simulink model "Vehicle_Powertrain_Trans_and_Controller_LIB"  (R2014a)
settings: Solver=ode45  StartTime=0.0  StopTime=10.0  RelTol=1e-3
undefined symbols (not defined in the file): clutchRise, p0, pressThresh
libraries: sdl_lib x7, fl_lib x6, nesl_utility x5
Description:
  | Copyright 2014 The MathWorks, Inc.
settings Model: Creator=smiller  LastModifiedBy=smiller
settings DataIOCC: SignalLoggingSaveFormat=ModelDataLogs
settings OptimizationCC: ExpressionDepthLimit=2147483647  InitFltsAndDblsToZero=on
settings DebuggingCC: UnderspecifiedInitializationDetection=Classic  FcnCallInpInsideContextMsg=UseLocalSettings  StateNameClashWarn=warning
settings SFSimCC: SimParseCustomCode=off
settings GRTTargetCC: CombineOutputUpdateFcns=off  GRTInterface=on

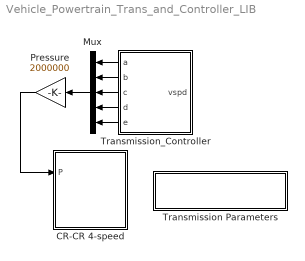
== system Vehicle_Powertrain_Trans_and_Controller_LIB ==
  CR-CR 4-speed : Subsystem  mask(CR-CR 4-Speed){}
      mask help: This is a template for a CR-CR 4-speed transmission. Copy it to your model, open it as a subsystem, and modify it for your use.
      mask init:
      | drive_preinitmask(); Icon = drive_crcrgearblock('Mask');
      settings: OpenFcn=open_system(gcbh,'force');
      mask Help: web(drive_help);
      mask Display:
      | plot(Icon.x1,Icon.y1);
      | plot(Icon.x1_1,Icon.y1_1);
      | plot(Icon.x2,Icon.y2);
      | plot(Icon.x3,Icon.y3);
      | plot(Icon.x3_1,Icon.y3_1);
      | plot(Icon.x4,Icon.y4);
      | plot(Icon.x5,Icon.y5);
      | plot(Icon.x6,Icon.y6);
      | plot(Icon.x7,Icon.y7);
      | plot(Icon.x8,Icon.y8);
      | plot(Icon.x9,Icon.y9);
      | plot(Icon.x10,Icon.y10);
      | plot(Icon.x11,Icon.y11);
      | plot(Icon.x12,Icon.y12);
      | plot(Icon.x13,Icon.y13);
      | plot(Icon.x14,Icon.y14);
      | plot(Icon.x15,Icon.y15);
      | plot(Icon.x16,Icon.y16);
      | plot(Icon.x16_1,Icon.y16_1);
      | plot(Icon.x16_2,Icon.y16_2);
      | plot(Icon.x17,Icon.y17);
      | plot(Icon.x18,Icon.y18);
      | plot(Icon.x18_1,Icon.y18_1);
      | plot(Icon.x18_2,Icon.y18_2);
      | plot(Icon.x19,Icon.y19);
      | plot(Icon.x20,Icon.y20);
      | plot(Icon.x21,Icon.y21);
      | plot(Icon.x22,Icon.y22);
      | plot(Icon.x23,Icon.y23);
      | plot(Icon.x24,Icon.y24);
      | plot(Icon.x25,Icon.y25);
      | plot(Icon.x26,Icon.y26);
      | plot(Icon.x27,Icon.y27);
      | plot(Icon.x28,Icon.y28);
      | plot(Icon.x29,Icon.y29);
      | 
      | plot(Icon.LowerLeftx,Icon.LowerLefty);
      | plot(Icon.UpperRightx,Icon.UpperRighty);
  Mux : Mux  Inputs=5
  Pressure : Gain  Gain=2000000
  Transmission Parameters : Subsystem
      settings: OpenFcn=|
      | num_fric_surf = 6;
      | eff_tor_rad = 0.4;
      | engagement_area = 0.0025;
      | peak_normal = 0.55;
      | fric_coeff = 0.5;
      | clutchRise = 0.1;
      | velTol = 1e-3;
      | pressThresh = 0.05;
      | p0 = 20e5;
      mask Display: fprintf('Double-Click to Define\nTransmission Parameters');
  Transmission_Controller : Stateflow chart  TreatAsAtomicUnit=on
  wires:
  Transmission_Controller/1(a) -> Mux/1
  Transmission_Controller/2(b) -> Mux/2
  Transmission_Controller/3(c) -> Mux/3
  Transmission_Controller/4(d) -> Mux/4
  Transmission_Controller/5(e) -> Mux/5
  Mux/1 -> Pressure/1
  Pressure/1 -> CR-CR 4-speed/1(P)

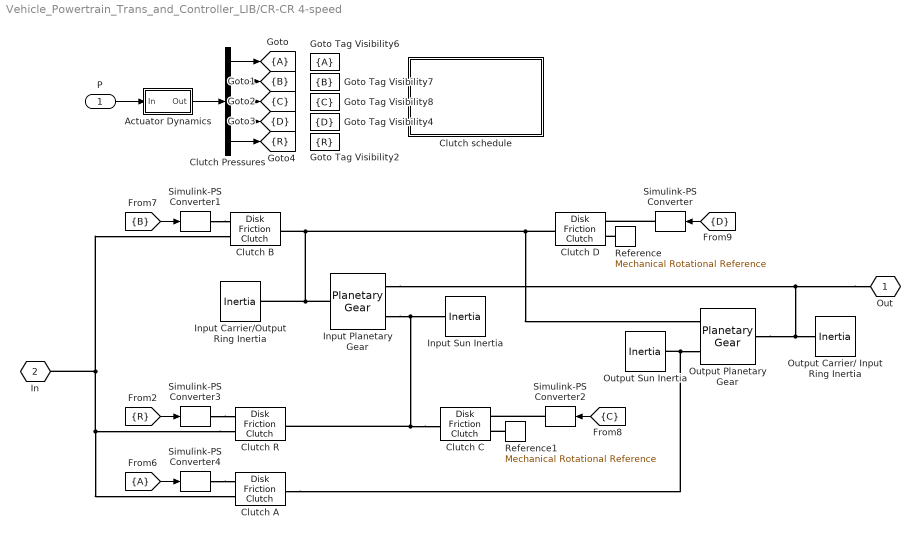
== system Vehicle_Powertrain_Trans_and_Controller_LIB/CR-CR 4-speed ==
  P : Inport
  Actuator Dynamics : Subsystem  mask(First-order lag supporting vector signals){b=clutchRise, x_initial=0}
      mask prompts: b "Filter time constant"; x_initial "Initial output"
      mask help: Models a lag of the form 1/(b*s+1) where s is the Laplace operator.
  Clutch Pressures : Demux  Outputs=5
  Clutch schedule : Subsystem
      mask Display: fprintf('Double-click to show\n Clutch Schedule')
  Clutch A : sdl_lib/Clutches/Disk Friction Clutch  geometry_model=1  r_eff=eff_tor_rad m  d_o=0.15 m  d_i=0.1 m  nS=num_fric_surf  piston_area=engagement_area m^2  friction_model=1  mu_coulomb=fric_coeff  mu_w_vector=[ 0 0.1 0.2 0.3 0.4 0.5 1 2 5 10 100 1000 ] rad/s  mu_coulomb_vector=[ 0.29 0.28 0.26 0.22 0.21 0.2 0.2 0.19 0.19 0.19 0.19 0.19 ]  mu_interp_method=1  mu_extrap_method=1  mu_static=peak_normal  d_f=1  w_tol=velTol rad/s  pressure_min=pressThresh*p0 Pa  mu_visc=0 N*m/(rad/s)  initial_state_locked=1
  Clutch B : sdl_lib/Clutches/Disk Friction Clutch  geometry_model=1  r_eff=eff_tor_rad m  d_o=0.15 m  d_i=0.1 m  nS=num_fric_surf  piston_area=engagement_area m^2  friction_model=1  mu_coulomb=fric_coeff  mu_w_vector=[ 0 0.1 0.2 0.3 0.4 0.5 1 2 5 10 100 1000 ] rad/s  mu_coulomb_vector=[ 0.29 0.28 0.26 0.22 0.21 0.2 0.2 0.19 0.19 0.19 0.19 0.19 ]  mu_interp_method=1  mu_extrap_method=1  mu_static=peak_normal  d_f=1  w_tol=velTol rad/s  pressure_min=pressThresh*p0 Pa  mu_visc=0 N*m/(rad/s)  initial_state_locked=0
  Clutch C : sdl_lib/Clutches/Disk Friction Clutch  geometry_model=1  r_eff=eff_tor_rad m  d_o=0.15 m  d_i=0.1 m  nS=num_fric_surf  piston_area=engagement_area m^2  friction_model=1  mu_coulomb=fric_coeff  mu_w_vector=[ 0 0.1 0.2 0.3 0.4 0.5 1 2 5 10 100 1000 ] rad/s  mu_coulomb_vector=[ 0.29 0.28 0.26 0.22 0.21 0.2 0.2 0.19 0.19 0.19 0.19 0.19 ]  mu_interp_method=1  mu_extrap_method=1  mu_static=peak_normal  d_f=1  w_tol=velTol rad/s  pressure_min=pressThresh*p0 Pa  mu_visc=0 N*m/(rad/s)  initial_state_locked=0
  Clutch D : sdl_lib/Clutches/Disk Friction Clutch  geometry_model=1  r_eff=eff_tor_rad m  d_o=0.15 m  d_i=0.1 m  nS=num_fric_surf  piston_area=engagement_area m^2  friction_model=1  mu_coulomb=fric_coeff  mu_w_vector=[ 0 0.1 0.2 0.3 0.4 0.5 1 2 5 10 100 1000 ] rad/s  mu_coulomb_vector=[ 0.29 0.28 0.26 0.22 0.21 0.2 0.2 0.19 0.19 0.19 0.19 0.19 ]  mu_interp_method=1  mu_extrap_method=1  mu_static=peak_normal  d_f=1  w_tol=velTol rad/s  pressure_min=pressThresh*p0 Pa  mu_visc=0 N*m/(rad/s)  initial_state_locked=1
  Clutch R : sdl_lib/Clutches/Disk Friction Clutch  geometry_model=1  r_eff=eff_tor_rad m  d_o=0.15 m  d_i=0.1 m  nS=num_fric_surf  piston_area=engagement_area m^2  friction_model=1  mu_coulomb=fric_coeff  mu_w_vector=[ 0 0.1 0.2 0.3 0.4 0.5 1 2 5 10 100 1000 ] rad/s  mu_coulomb_vector=[ 0.29 0.28 0.26 0.22 0.21 0.2 0.2 0.19 0.19 0.19 0.19 0.19 ]  mu_interp_method=1  mu_extrap_method=1  mu_static=peak_normal  d_f=1  w_tol=velTol rad/s  pressure_min=pressThresh*p0 Pa  mu_visc=0 N*m/(rad/s)  initial_state_locked=0
  Goto Tag Visibility2 : GotoTagVisibility  GotoTag=R
  Goto Tag Visibility4 : GotoTagVisibility  GotoTag=D
  Goto Tag Visibility6 : GotoTagVisibility
  Goto Tag Visibility7 : GotoTagVisibility  GotoTag=B
  Goto Tag Visibility8 : GotoTagVisibility  GotoTag=C
  "Input Planetary Gear " : sdl_lib/Gears/Planetary Gear  rs_ratio=2.2258  friction_model=1  efficiency=[ 0.96 0.98 ]  mu_visc=[ 0 0 ] N*m/(rad/s)  w_thr=[ 0.01 0.01 ] rad/s
  Input Carrier/Output Ring Inertia : fl_lib/Mechanical/Rotational Elements/Inertia  inertia=1e-4 kg*m^2  w_specify=on  w_priority=High  w=0 rad/s  t_specify=off  t_priority=High  t=0 N*m
  Input Sun Inertia : fl_lib/Mechanical/Rotational Elements/Inertia  inertia=1e-4 kg*m^2  w_specify=on  w_priority=High  w=0 rad/s  t_specify=off  t_priority=High  t=0 N*m
  Output Planetary Gear : sdl_lib/Gears/Planetary Gear  rs_ratio=1.84  friction_model=1  efficiency=[ 0.96 0.98 ]  mu_visc=[0 0] N*m/(rad/s)  w_thr=[ 0.01 0.01 ] rad/s
  "Output Carrier/ Input Ring Inertia " : fl_lib/Mechanical/Rotational Elements/Inertia  inertia=1e-4 kg*m^2  w_specify=on  w_priority=High  w=0 rad/s  t_specify=off  t_priority=High  t=0 N*m
  Output Sun Inertia : fl_lib/Mechanical/Rotational Elements/Inertia  inertia=1e-4 kg*m^2  w_specify=on  w_priority=High  w=0 rad/s  t_specify=off  t_priority=High  t=0 N*m
  Reference : fl_lib/Mechanical/Rotational Elements/Mechanical Rotational Reference
  Reference1 : fl_lib/Mechanical/Rotational Elements/Mechanical Rotational Reference
  Simulink-PS Converter{,1..4} (5 alike) : nesl_utility/Simulink-PS Converter  PhysicalDomain=network_engine_domain  SubClassName=ps_input  LeftPortType=input  RightPortType=output  PseudoPeriodic=off  Frequencies=[]  NoiseDistribution=none  NoiseParameters=[]  Unit=1  AffineConversion=off  InputFiltering=off  SimscapeFilterOrder=1  InputFilterTimeConstant=.001  UdotUserProvided=0
  Out : PMIOPort  Tag=PMCPort  Port=1  Side=Right
  In : PMIOPort  Tag=PMCPort  Port=2  Side=Left
  tag scope: A=scoped, B=scoped, C=scoped, D=scoped, R=scoped
  wires:
  [A] -> Simulink-PS Converter4/1
  [R] -> Simulink-PS Converter3/1
  [C] -> Simulink-PS Converter2/1
  [B] -> Simulink-PS Converter1/1
  [D] -> Simulink-PS Converter/1
  Clutch Pressures/5 -> [R]
  Clutch Pressures/4 -> [D]
  Clutch Pressures/3 -> [C]
  Clutch Pressures/2 -> [B]
  Clutch Pressures/1 -> [A]
  P/1 -> Actuator Dynamics/1(In)
  Actuator Dynamics/1(Out) -> Clutch Pressures/1
  connections:
  Simulink-PS Converter4/RConn1 -- Clutch A/LConn1
  Simulink-PS Converter3/RConn1 -- Clutch R/LConn1
  Simulink-PS Converter2/RConn1 -- Clutch C/LConn1
  Reference1/LConn1 -- Clutch C/LConn2
  Clutch R/LConn2 -- Clutch B/LConn2 -- In/RConn1 -- Clutch A/LConn2
  Simulink-PS Converter1/RConn1 -- Clutch B/LConn1
  Input Carrier/Output Ring Inertia/LConn1 -- "Input Planetary Gear "/LConn1 -- Clutch D/RConn1 -- Output Planetary Gear/RConn1 -- Clutch B/RConn1
  Clutch C/RConn1 -- Input Sun Inertia/LConn1 -- "Input Planetary Gear "/RConn2 -- Clutch R/RConn1
  Simulink-PS Converter/RConn1 -- Clutch D/LConn1
  Reference/LConn1 -- Clutch D/LConn2
  Output Sun Inertia/LConn1 -- Output Planetary Gear/RConn2 -- Clutch A/RConn1
  Out/RConn1 -- "Output Carrier/ Input Ring Inertia "/LConn1 -- Output Planetary Gear/LConn1 -- "Input Planetary Gear "/RConn1

== system Vehicle_Powertrain_Trans_and_Controller_LIB/Transmission Parameters ==

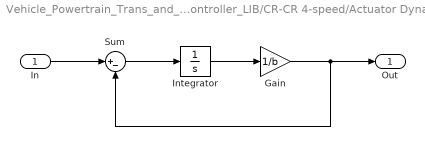
== system Vehicle_Powertrain_Trans_and_Controller_LIB/CR-CR 4-speed/Actuator Dynamics ==
  In : Inport
  Gain : Gain  Gain=1/b
  Integrator : Integrator  InitialCondition=x_initial
  Sum : Sum  Inputs=|+-  SaturateOnIntegerOverflow=on  InputSameDT=on  OutDataTypeStr=Inherit: Same as first input
  Out : Outport
  wires:
  Sum/1 -> Integrator/1
  In/1 -> Sum/1
  Integrator/1 -> Gain/1
  Gain/1 -> Sum/2, Out/1

== system Vehicle_Powertrain_Trans_and_Controller_LIB/CR-CR 4-speed/Clutch schedule ==
  note: ---------------------------------------------------------------------------------------------------------------------------------------------------------------
  note: ---------------------------------------------------------------------------------------------------------------------------------------------------------------
  note: ---------------------------------------------------------------------------------------------------------------------------------------------------------------
  note: ---------------------------------------------------------------------------------------------------------------------------------------------------------------
  note: |
      | |
      | |
      | |
      | |
      | |
      | |
      | |
      | |
      | |
      | |
      | |
      | |
      | |
  note: ---------------------------------------------------------------------------------------------------------------------------------------------------------------
  note: ---------------------------------------------------------------------------------------------------------------------------------------------------------------
  note: |
      | |
      | |
      | |
      | |
      | |
      | |
      | |
      | |
      | |
      | |
      | |
      | |
      | |
  note: |
      | |
      | |
      | |
      | |
      | |
      | |
      | |
      | |
      | |
      | |
      | |
      | |
      | |
  note: |
      | |
      | |
      | |
      | |
      | |
      | |
      | |
      | |
      | |
      | |
      | |
      | |
      | |
  note: |
      | |
      | |
      | |
      | |
      | |
      | |
      | |
      | |
      | |
      | |
      | |
      | |
      | |
  note: |
      | |
      | |
      | |
      | |
      | |
      | |
      | |
      | |
      | |
      | |
      | |
      | |
      | |
  note: |
      | |
      | |
      | |
      | |
      | |
      | |
      | |
      | |
      | |
      | |
      | |
      | |
      | |
  note: |
      | |
      | |
      | |
      | |
      | |
      | |
      | |
      | |
      | |
      | |
      | |
      | |
      | |
  note: ---------------------------------------------------------------------------------------------------------------------------------------------------------------
  note: g1/(1+g1)
  note: 1
  note: (g1+g2)/(1+g1)
  note: g2
  note: -g1
  note: F
  note: L
  note: F
  note: L
  note: L
  note: F
  note: L
  note: L
  note: L
  note: F
  note: F
  note: F
  note: L
  note: F
  note: L
  note: Ratio
  note: L
  note: F
  note: F
  note: F
  note: R
      |
      | 1
      |
      | 2
      |
      | 3
      |
      | 4
  note: Clutch Schedule
  note: Gear
  note: A
  note: B
  note: C
  note: D
  note: E
  note: L
  note: F
  note: F
  note: F
  note: F
  note: F
  note: g1: Ravigneaux ring (R)/large sun (S1) gear ratio
      | g2: Ravigneaux ring (R)/small sun (S2) gear ratio
  note: F = Free
      | L = Locked

== stateflow chart Vehicle_Powertrain_Trans_and_Controller_LIB/Transmission_Controller ==
  state first
    a=0;
    b=0;
    c=0;
    d=0;
    e=0;
  state third
    a=0;
    b=0;
    c=0;
    d=0;
    e=0;
  state second
    a=0;
    b=0;
    c=0;
    d=0;
    e=0;
  state fourth
    a=0;
    b=0;
    c=0;
    d=0;
    e=0;
  third -> fourth [order 1] : [vspd>100]
  first -> second : [vspd>30]
  second -> third [order 1] : [vspd>65]
  (default) -> first
  second -> first [order 2] : [vspd<20]
  third -> second [order 2] : [vspd<55]
  fourth -> third : [vspd<90]
  data: vspd input; a output double; b output double; c output double; d output double; e output double
